simulink model "heli_q8_d3p3"  (R2015b)
settings: Solver=ode1  StartTime=0.0  StopTime=inf  FixedStep=0.002  RelTol=1e-3
PostLoadFcn:
  | qc_set_target_type(getConfigSet(bdroot, 'QUARC Default Target Configuration'));
values from neighbouring files (symbols this model uses):
  F = [0 2*K(1,3); 2*K(2,1) 0]    [Dag3p3.m]
  Joystick_gain_x = 3    [init_heli_d3p3.m]
  Joystick_gain_y = 6    [init_heli_d3p3.m]
  K = lqr(A, B, Q, R)    [Dag3p3.m]
  V_s0 = 7.0    (= 7)    [init_heli_d3p3.m]
undefined symbols (not defined in the file or in its folder): HIL, qc_get_step_size
libraries: quarc_library x4
settings Model: SimulationMode=external  ExtModeTrigDuration=5000  Creator=Rchan  LastModifiedBy=jahnpn
settings SolverCC: PositivePriorityOrder=on
settings DataIOCC: SaveFormat=Array  SignalLoggingSaveFormat=ModelDataLogs
settings OptimizationCC: ExpressionDepthLimit=2147483647  InitFltsAndDblsToZero=on
settings DebuggingCC: SaveWithParameterizedLinksMsg=none  UnderspecifiedInitializationDetection=Classic  MergeDetectMultiDrivingBlocksExec=none  SolverPrmCheckMsg=warning  MultiTaskDSMMsg=warning  MultiTaskCondExecSysMsg=none  FcnCallInpInsideContextMsg=UseLocalSettings  StateNameClashWarn=warning
settings HardwareCC: ProdBitPerPointer=32  ProdLargestAtomicFloat=None  ProdIntDivRoundTo=Undefined  ProdEndianess=Unspecified  ProdWordSize=32  ProdHWDeviceType=32-bit Generic
settings RTWCC: SystemTargetFile=quarc_win64.tlc  TemplateMakefile=quarc_default_tmf  Description=QUARC Win64 Target
settings GRTTargetCC: ParMdlRefBuildCompliant=off  CompOptLevelCompliant=off  GeneratePreprocessorConditionals=Disable all  CombineOutputUpdateFcns=off  MatFileLogging=off  GRTInterface=on  UseToolchainInfoCompliant=off  ExtMode=on  ExtModeMexFile=quarc_comm
settings ConfigComp: CovModelRefEnable=Off  CovSFcnEnable=off

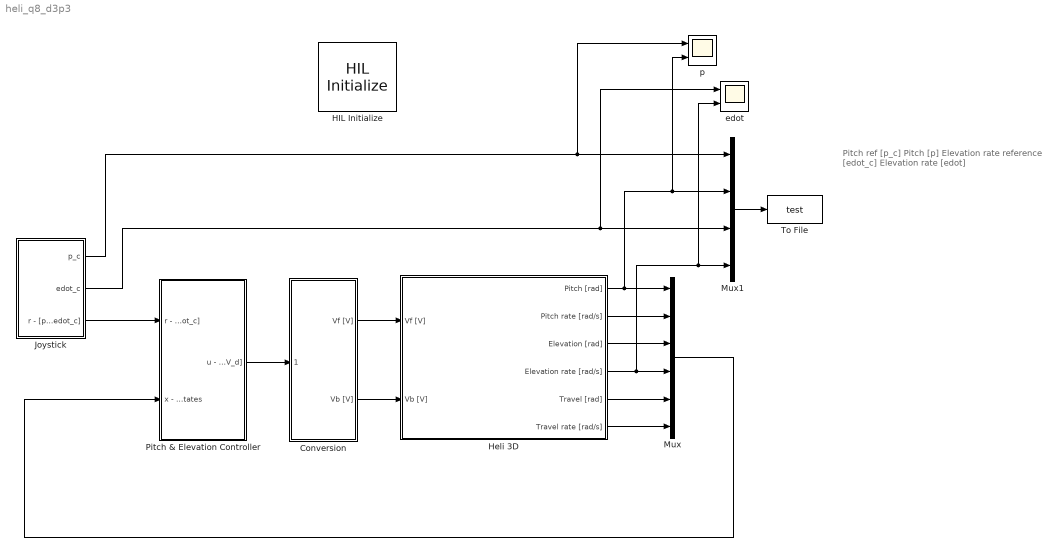
== system heli_q8_d3p3 ==
  note: Pitch ref [p_c]
      |
      |
      | Pitch [p]
      |
      |
      | Elevation rate reference [edot_c]
      |
      |
      | Elevation rate [edot]
  Conversion : Subsystem
  HIL Initialize : quarc_library/Data Acquisition/Generic/Configuration/HIL Initialize  Priority=-99  object_name=HIL-1  board_type=q8_usb  board_number=0  board_options=update_rate=normal;decimation=1  exclusive=off  active=off  hardware_clocks=[0:2]  clock_modes=[]  initial_clock_frequencies=[]  set_clock_params_at_start=off  set_clock_params_at_switch_in=off  set_clock_frequencies_at_start=off  set_clock_frequencies_at_switch_in=off  analog_input_channels=[0:7]  analog_input_maximums=10  analog_input_minimums=-10  set_analog_input_params_at_start=on  set_analog_input_params_at_switch_in=off  analog_output_channels=[0:7]  analog_output_maximums=10  analog_output_minimums=-10  initial_analog_outputs=[0]  final_analog_outputs=[0]  watchdog_analog_outputs=0  set_analog_output_params_at_start=on  set_analog_output_params_at_switch_in=off  set_analog_outputs_at_start=on  set_analog_outputs_at_switch_in=off  set_analog_outputs_at_terminate=on  set_analog_outputs_at_switch_out=off  set_analog_outputs_on_watchdog=off  digital_input_channels=[]  digital_output_channels=[]  digital_output_configuration=[]  initial_digital_outputs=[1]  final_digital_outputs=[1]  watchdog_digital_outputs=[1]  set_digital_output_params_at_start=off  set_digital_output_params_at_switch_in=off  set_digital_outputs_at_start=on  set_digital_outputs_at_switch_in=off  set_digital_outputs_at_terminate=on  set_digital_outputs_at_switch_out=off  set_digital_outputs_on_watchdog=off  encoder_channels=[0:7]  quadrature=[4]  encoder_filter_frequency=[]  initial_encoder_counts=[0]  set_encoder_params_at_start=on  set_encoder_params_at_switch_in=off  set_encoder_counts_at_start=on  set_encoder_counts_at_switch_in=off  pwm_channels=[0:7]  pwm_modes=0  pwm_frequency=99.532799999999995e6/4095  pwm_configuration=[0]  pwm_alignment=[0]  pwm_polarity=[1]  pwm_leading_deadband=[0]  pwm_trailing_deadband=[0]  initial_pwm_outputs=[0]  final_pwm_outputs=[0]  watchdog_pwm_outputs=[0]  set_pwm_params_at_start=on  set_pwm_params_at_switch_in=off  set_pwm_outputs_at_start=on  set_pwm_outputs_at_switch_in=off  set_pwm_outputs_at_terminate=on  set_pwm_outputs_at_switch_out=off  set_pwm_outputs_on_watchdog=off  other_output_channels=[]  initial_other_outputs=[]  final_other_outputs=[]  watchdog_other_outputs=[]  set_other_outputs_at_start=off  set_other_outputs_at_switch_in=off  set_other_outputs_at_terminate=off  set_other_outputs_at_switch_out=off  set_other_outputs_on_watchdog=off
  Heli 3D : Subsystem
  Joystick : Subsystem
  Mux : Mux  Inputs=6
  Mux1 : Mux
  Pitch & Elevation Controller : Subsystem
  To File : ToFile  Filename=test  MatrixName=test
  edot : Scope  NumInputPorts=2
  p : Scope  NumInputPorts=2
  wires:
  Conversion/2(Vb [V]) -> Heli 3D/2(Vb [V])
  Conversion/1(Vf [V]) -> Heli 3D/1(Vf [V])
  Mux/1 -> Pitch & Elevation Controller/2(x - 6 states)
  Mux1/1 -> To File/1
  Pitch & Elevation Controller/1("u - [V_s, V_d]") -> Conversion/1(u - [Vs,Vd])
  Heli 3D/6(Travel rate [rad/s]) -> Mux/6
  Heli 3D/5(Travel [rad]) -> Mux/5
  Heli 3D/4(Elevation rate [rad/s]) -> Mux/4, edot/2, Mux1/4
  Heli 3D/3(Elevation [rad]) -> Mux/3
  Heli 3D/2(Pitch rate [rad/s]) -> Mux/2
  Heli 3D/1(Pitch [rad]) -> p/2, Mux1/2, Mux/1
  Joystick/3("r - [p_c, edot_c]") -> Pitch & Elevation Controller/1("r - [p_c, edot_c]")
  Joystick/2(edot_c) -> edot/1, Mux1/3
  Joystick/1(p_c) -> p/1, Mux1/1

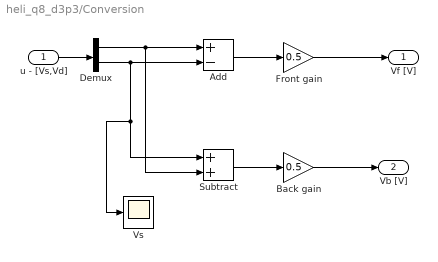
== system heli_q8_d3p3/Conversion ==
  u - [Vs,Vd] : Inport
  Add : Sum  Inputs=+-
  Back gain : Gain  Gain=0.5
  Demux : Demux  Outputs=2
  Front gain : Gain  Gain=0.5
  Subtract : Sum
  Vs : Scope
  Vf [V] : Outport
  Vb [V] : Outport  Port=2
  wires:
  Demux/2 -> Vs/1, Subtract/1, Add/2
  Subtract/1 -> Back gain/1
  Back gain/1 -> Vb [V]/1
  Add/1 -> Front gain/1
  Front gain/1 -> Vf [V]/1
  Demux/1 -> Add/1, Subtract/2
  u - [Vs,Vd]/1 -> Demux/1

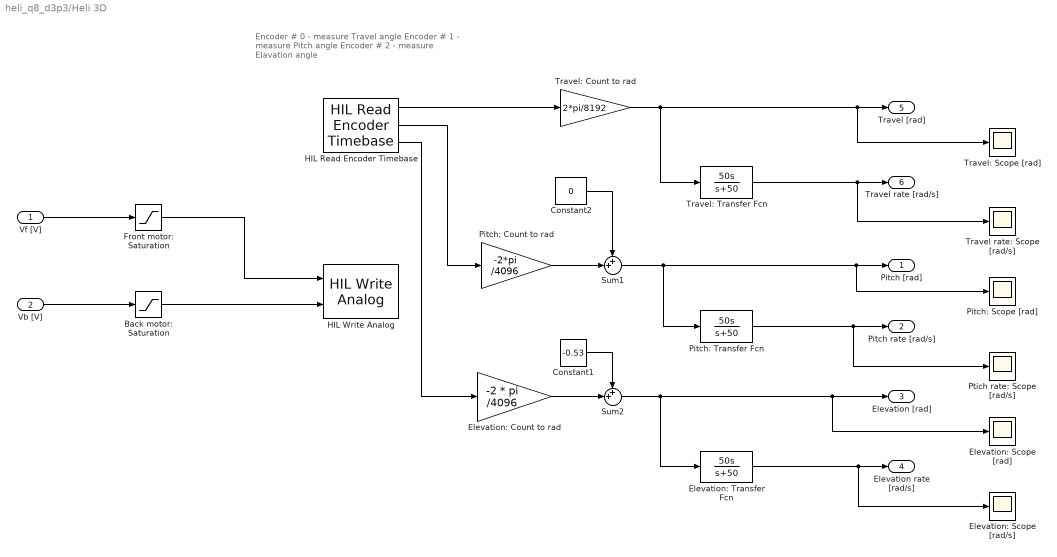
== system heli_q8_d3p3/Heli 3D ==
  note: Encoder # 0 - measure Travel angle
      | Encoder # 1 - measure Pitch angle
      | Encoder # 2 - measure Elavation angle
  Vf [V] : Inport
  Vb [V] : Inport  Port=2
  Back motor: Saturation : Saturate  UpperLimit=5  LowerLimit=-5
  Constant1 : Constant  Value=-0.53
  Constant2 : Constant  Value=0
  Elevation: Count to rad : Gain  Gain=-2 * pi /4096
  Elevation: Scope [rad/s] : Scope
  Elevation: Scope [rad] : Scope
  Elevation: Transfer Fcn : TransferFcn  Numerator=[50 0]  Denominator=[1 50]
  Front motor: Saturation : Saturate  UpperLimit=5  LowerLimit=-5
  HIL Read Encoder Timebase : quarc_library/Data Acquisition/Generic/Timebases/HIL Read Encoder Timebase  object_name=HIL-1  clock=0  channels=[0:2]  samples_in_buffer=max(ceil(1/qc_get_step_size), 1)  active=on  vector_output=off  data_type_mode=Inherit via back propagation  data_type=double
  HIL Write Analog : quarc_library/Data Acquisition/Generic/Immediate I//O/HIL Write Analog  object_name=HIL-1  channels=[0:1]  sample_time=-1  active=off  vector_input=off
  Pitch: Count to rad : Gain  Gain=-2*pi /4096
  Pitch: Scope [rad] : Scope
  Pitch: Transfer Fcn : TransferFcn  Numerator=[50 0]  Denominator=[1 50]
  Ptich rate: Scope [rad/s] : Scope
  Sum1 : Sum  Inputs=++|
  Sum2 : Sum  Inputs=++|
  Travel rate: Scope [rad/s] : Scope
  Travel: Count to rad : Gain  Gain=2*pi/8192
  Travel: Scope [rad] : Scope
  Travel: Transfer Fcn : TransferFcn  Numerator=[50 0]  Denominator=[1 50]
  Pitch [rad] : Outport
  Pitch rate [rad/s] : Outport  Port=2
  Elevation [rad] : Outport  Port=3
  Elevation rate [rad/s] : Outport  Port=4
  Travel [rad] : Outport  Port=5
  Travel rate [rad/s] : Outport  Port=6
  wires:
  Travel: Count to rad/1 -> Travel: Scope [rad]/1, Travel [rad]/1, Travel: Transfer Fcn/1
  Travel: Transfer Fcn/1 -> Travel rate: Scope [rad/s]/1, Travel rate [rad/s]/1
  Pitch: Transfer Fcn/1 -> Ptich rate: Scope [rad/s]/1, Pitch rate [rad/s]/1
  Elevation: Transfer Fcn/1 -> Elevation: Scope [rad/s]/1, Elevation rate [rad/s]/1
  Vf [V]/1 -> Front motor: Saturation/1
  Vb [V]/1 -> Back motor: Saturation/1
  Front motor: Saturation/1 -> HIL Write Analog/1
  Back motor: Saturation/1 -> HIL Write Analog/2
  HIL Read Encoder Timebase/1 -> Travel: Count to rad/1
  HIL Read Encoder Timebase/3 -> Elevation: Count to rad/1
  Elevation: Count to rad/1 -> Sum2/2
  Constant1/1 -> Sum2/1
  Sum2/1 -> Elevation: Scope [rad]/1, Elevation [rad]/1, Elevation: Transfer Fcn/1
  Constant2/1 -> Sum1/1
  Pitch: Count to rad/1 -> Sum1/2
  Sum1/1 -> Pitch: Transfer Fcn/1, Pitch: Scope [rad]/1, Pitch [rad]/1
  HIL Read Encoder Timebase/2 -> Pitch: Count to rad/1

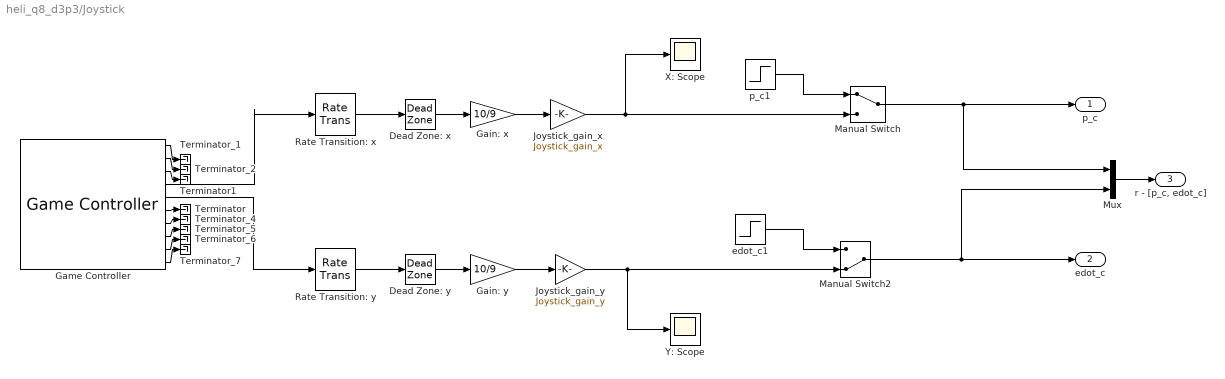
== system heli_q8_d3p3/Joystick ==
  Dead Zone: x : DeadZone  LowerValue=-0.1  UpperValue=0.1  SaturateOnIntegerOverflow=on
  Dead Zone: y : DeadZone  LowerValue=-0.1  UpperValue=0.1  SaturateOnIntegerOverflow=on
  Gain: x : Gain  Gain=10/9
  Gain: y : Gain  Gain=10/9
  Game Controller : quarc_library/Devices/Peripherals/Target/Game Controller  controller=1  buffer_size=12  deadzone=[]  saturation=[]  sample_time=max(qc_get_step_size, 0.01)  auto_center=off  enabled=on
  Joystick_gain_x : Gain  Gain=Joystick_gain_x
  Joystick_gain_y : Gain  Gain=Joystick_gain_y
  Manual Switch : ManualSwitch
  Manual Switch2 : ManualSwitch  CurrentSetting=0
  Mux : Mux  Inputs=2
  Rate Transition: x : RateTransition
  Rate Transition: y : RateTransition
  Terminator : Terminator
  Terminator1 : Terminator
  Terminator_{1..2,4..7} (6 alike) : Terminator
  X: Scope : Scope
  Y: Scope : Scope
  edot_c1 : Step  Time=5  Before=-0.1  After=0.3  SampleTime=0
  p_c1 : Step  Time=5  Before=-0.2  After=0.4  SampleTime=0
  p_c : Outport
  edot_c : Outport  Port=2
  "r - [p_c, edot_c]" : Outport  Port=3
  wires:
  Rate Transition: y/1 -> Dead Zone: y/1
  Rate Transition: x/1 -> Dead Zone: x/1
  Game Controller/5 -> Rate Transition: y/1
  Game Controller/4 -> Rate Transition: x/1
  Game Controller/1 -> Terminator_1/1
  Game Controller/2 -> Terminator_2/1
  Game Controller/7 -> Terminator_4/1
  Game Controller/8 -> Terminator_5/1
  Game Controller/9 -> Terminator_6/1
  Game Controller/10 -> Terminator_7/1
  Game Controller/3 -> Terminator1/1
  Game Controller/6 -> Terminator/1
  Dead Zone: x/1 -> Gain: x/1
  Dead Zone: y/1 -> Gain: y/1
  Gain: x/1 -> Joystick_gain_x/1
  Gain: y/1 -> Joystick_gain_y/1
  Joystick_gain_x/1 -> Manual Switch/2, X: Scope/1
  Joystick_gain_y/1 -> Manual Switch2/2, Y: Scope/1
  Mux/1 -> "r - [p_c, edot_c]"/1
  edot_c1/1 -> Manual Switch2/1
  p_c1/1 -> Manual Switch/1
  Manual Switch2/1 -> edot_c/1, Mux/2
  Manual Switch/1 -> Mux/1, p_c/1

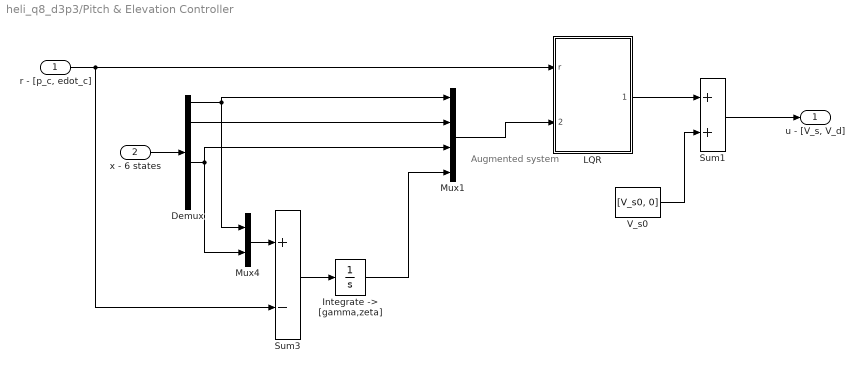
== system heli_q8_d3p3/Pitch & Elevation Controller ==
  note: Augmented
      | system
  "r - [p_c, edot_c]" : Inport
  x - 6 states : Inport  Port=2
  Demux : Demux  Outputs=6
  "Integrate -> [gamma,zeta]" : Integrator
  LQR : Subsystem
  Mux1 : Mux
  Mux4 : Mux  Inputs=2
  Sum1 : Sum  SaturateOnIntegerOverflow=on  InputSameDT=on  OutDataTypeStr=Inherit: Same as first input
  Sum3 : Sum  Inputs=+-  SaturateOnIntegerOverflow=on  InputSameDT=on  OutDataTypeStr=Inherit: Same as first input
  V_s0 : Constant  Value=[V_s0, 0]
  "u - [V_s, V_d]" : Outport
  wires:
  Sum1/1 -> "u - [V_s, V_d]"/1
  "r - [p_c, edot_c]"/1 -> Sum3/2, LQR/1(r)
  V_s0/1 -> Sum1/2
  LQR/1("[~V_s,V_d]") -> Sum1/1
  x - 6 states/1 -> Demux/1
  Demux/1 -> Mux1/1, Mux4/1
  Demux/2 -> Mux1/2
  Demux/4 -> Mux4/2, Mux1/3
  Mux1/1 -> LQR/2(x - 5 states)
  Sum3/1 -> "Integrate -> [gamma,zeta]"/1
  Mux4/1 -> Sum3/1
  "Integrate -> [gamma,zeta]"/1 -> Mux1/4

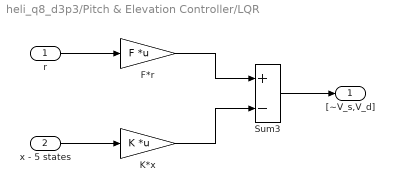
== system heli_q8_d3p3/Pitch & Elevation Controller/LQR ==
  r : Inport
  x - 5 states : Inport  Port=2
  F*r : Gain  Gain=F  Multiplication=Matrix(K*u)
  K*x : Gain  Gain=K  Multiplication=Matrix(K*u)
  Sum3 : Sum  Inputs=+-  SaturateOnIntegerOverflow=on  InputSameDT=on  OutDataTypeStr=Inherit: Same as first input
  "[~V_s,V_d]" : Outport  InitialOutput=0
  wires:
  Sum3/1 -> "[~V_s,V_d]"/1
  r/1 -> F*r/1
  x - 5 states/1 -> K*x/1
  F*r/1 -> Sum3/1
  K*x/1 -> Sum3/2
